simulink model "thruster"  (R2023a)
settings: Solver=ode4  StartTime=0.0  StopTime=10.0  FixedStep=dt  RelTol=1e-3
libraries: vrlib x1
settings Model: Creator=ndelurgio  LastModifiedBy=ndelurgio

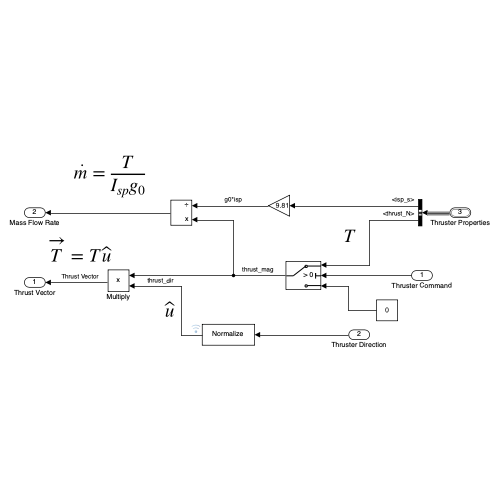
[thumbnail: Simulink's stored preview of the top-level diagram]
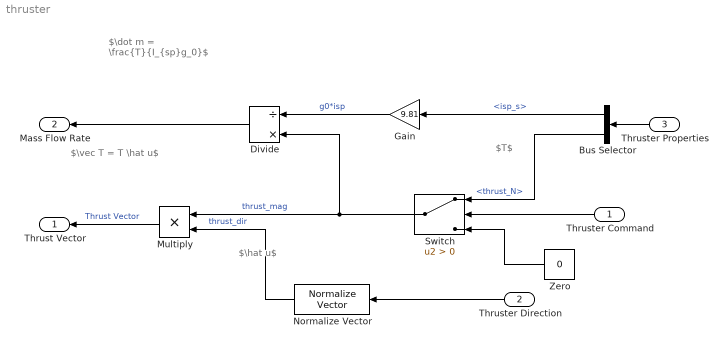
== system thruster ==
  note: $\dot m = \frac{T}{I_{sp}g_0}$
  note: $\vec T = T \hat u$
  note: $\hat u$
  note: $T$
  Thruster Command : Inport
  Thruster Direction : Inport  Port=2  PortDimensions=3
  Thruster Properties : Inport  Port=3  OutDataTypeStr=Bus: thruster
  Bus Selector : BusSelector  OutputSignals=isp_s,thrust_N
  Divide : Product  Inputs=/*
  Gain : Gain  Gain=9.81
  Multiply : Product  Inputs=**
  Normalize Vector : vrlib/Utilities/Normalize Vector  maxzero=0
  Switch : Switch  Criteria=u2 > Threshold  SaturateOnIntegerOverflow=off  InputSameDT=off
  Zero : Constant  Value=0  OutDataTypeStr=Inherit: Inherit via back propagation
  Thrust Vector : Outport  PortDimensions=3
  Mass Flow Rate : Outport  Port=2
  wires:
  Thruster Command/1 -> Switch/2
  Zero/1 -> Switch/3
  Thruster Properties/1 -> Bus Selector/1
  Switch/1 -> Divide/2, Multiply/1  "thrust_mag"
  Normalize Vector/1 -> Multiply/2  "thrust_dir"
  Multiply/1 -> Thrust Vector/1  "Thrust Vector"
  Bus Selector/2 -> Switch/1  "<thrust_N>"
  Bus Selector/1 -> Gain/1  "<isp_s>"
  Gain/1 -> Divide/1  "g0*isp"
  Divide/1 -> Mass Flow Rate/1
  Thruster Direction/1 -> Normalize Vector/1
